simulink model "gm_soc_dvbs2_fpga"  (R2025b)
settings: Solver=VariableStepAuto  StartTime=0.0  StopTime=10.0  RelTol=1e-3
InitFcn:
  | soc_dvbs2_init;
undefined symbols (not defined in the file or in its folder): Add, coefficientsLog, coefficientsSqrt1, coefficientsSqrt2, dataBits, Deinterleaver, designMultirateFIR, noisePow, Shift, Short, soc_dvbs2_designFIRFilter, soc_dvbs2_txPacketBits, syncWord, txDataOut, txFiltCoeff, XData
libraries: simulink x304, hdlsllib x265, dspsigops x15, dsphdlfiltering2 x8, hdlmdlgenlib x6, dsphdlsigops2 x5, commseqgen3 x5, dsphdlmathfun2 x3, hwlogicconnlib x2, whdledac x2, commhdlcrc x2, whdlutilities x1
(part 34 of 36)

== system gm_soc_dvbs2_fpga/DVBS2/DVBS2 TxRx/DVB-S2 HDL Receiver/Synchronizer and PL Header Decoder/Time Frequency and Coarse Phase Synchronizer/Fine Frequency Synchronizer/Modified L and R Algorithm/L and R Algorithm 18 point/Compute R(m) for 1 to 6/Compute R(m)_1 ==
  z : Inport  OutDataTypeStr=fixdt(1, 16, 11)  PortDimensions=1  SampleTime=2.5e-07
      settings: SignalType=complex
  zvalid : Inport  Port=2  OutDataTypeStr=boolean  PortDimensions=1  SampleTime=2.5e-07
  Add3 : Sum  OutDataTypeStr=fixdt(1, 33, 22)  AccumDataTypeStr=fixdt(1, 34, 22)  SampleTime=2.5e-07
  Compare To Constant : simulink/Logic and Bit Operations/Compare To Constant  relop=>=  const="fi(0,0,6,0,\"hex\",\"01\")"  OutDataTypeStr=boolean
  Compare To Constant2 : simulink/Logic and Bit Operations/Compare To Constant  relop===  const="fi(0,0,6,0,\"hex\",\"23\")"  OutDataTypeStr=boolean
  Complex Multiplier : Subsystem
  Delay{,1..2,7..9,11..12,14..15} (10 alike) : Delay  DelayLength=double(1)  InitialCondition=0  SampleTime=2.5e-07
  Delay{3..6,10,13,16..26} (17 alike) : Delay  DelayLength=double(2)  InitialCondition=0  SampleTime=2.5e-07
  Delay{27..30} (4 alike) : Delay  DelayLength=double(8)  InitialCondition=0  SampleTime=2.5e-07
  Gain : Gain  Gain="fi(0,0,16,21,\"hex\",\"ea0f\")"  ParamDataTypeStr=fixdt(0, 16, 21)  OutDataTypeStr=fixdt(1, 33, 22)  SampleTime=2.5e-07
  HDL Counter : hdlsllib/Sources/HDL Counter  CountType=Count limited  CountInit=0  CountStep=1  CountMax=N-1  CountFromType=Initial value  CountFrom=0  CountResetPort=off  CountLoadPort=off  CountEnbPort=on  CountDirPort=off  CountHitOutputPort=off  CountDataType=Unsigned  CountWordLen=nextpow2(N-1)  CountFracLen=0  CountSampTime=1
  Logical Operator : Logic  AllPortsSameDT=off  OutDataTypeStr=boolean  SampleTime=2.5e-07
  Logical Operator1 : Logic  AllPortsSameDT=off  OutDataTypeStr=boolean  SampleTime=2.5e-07
  Math Function : Math  Operator=conj  OutDataTypeStr=fixdt(1, 16, 11)
  Unit Delay Enabled Resettable Synchronous : hdlsllib/Discrete/Unit Delay Enabled Resettable Synchronous  InitialCondition=double(0)  SampleTime=-1
  Unit Delay Enabled Synchronous : hdlsllib/Discrete/Unit Delay Enabled Synchronous  InitialCondition=double(0)  SampleTime=-1
  Out1 : Outport  SampleTime=2.5e-07
  wires:
  zvalid/1 -> Delay14/1
  Logical Operator1/1 -> Delay23/1
  Delay10/1 -> Delay27/1
  Delay21/1 -> Gain/1
  Delay14/1 -> Delay15/1, HDL Counter/1, Delay9/1
  Delay9/1 -> Delay10/1
  HDL Counter/1 -> Delay12/1, Delay11/1
  Delay11/1 -> Delay5/1
  Delay22/1 -> Add3/2
  Delay15/1 -> Delay16/1
  z/1 -> Delay2/1
  Delay12/1 -> Delay6/1
  Delay16/1 -> Delay30/1
  Delay2/1 -> Delay7/1, Delay/1
  Delay27/1 -> Delay17/1
  Delay5/1 -> Delay28/1
  Delay6/1 -> Delay29/1
  Complex Multiplier/1(Out1) -> Delay13/1
  Delay7/1 -> Delay3/1
  Delay/1 -> Math Function/1
  Delay28/1 -> Compare To Constant/1
  Delay29/1 -> Compare To Constant2/1
  Delay30/1 -> Delay20/1
  Delay19/1 -> Logical Operator/1
  Math Function/1 -> Delay8/1
  Delay1/1 -> Unit Delay Enabled Synchronous/2, Unit Delay Enabled Resettable Synchronous/3
  Delay17/1 -> Logical Operator1/1
  Delay13/1 -> Delay21/1
  Compare To Constant2/1 -> Delay19/1
  Compare To Constant/1 -> Delay18/1
  Delay3/1 -> Complex Multiplier/1(In1)
  Delay8/1 -> Delay4/1
  Delay18/1 -> Logical Operator1/2
  Delay20/1 -> Logical Operator/2
  Delay4/1 -> Complex Multiplier/2(In2)
  Logical Operator/1 -> Delay25/1
  Delay24/1 -> Unit Delay Enabled Resettable Synchronous/2
  Delay23/1 -> Delay24/1
  Delay25/1 -> Delay26/1
  Delay26/1 -> Delay1/1
  Gain/1 -> Delay22/1
  Unit Delay Enabled Resettable Synchronous/1 -> Unit Delay Enabled Synchronous/1, Add3/1
  Unit Delay Enabled Synchronous/1 -> Out1/1
  Add3/1 -> Unit Delay Enabled Resettable Synchronous/1

== system gm_soc_dvbs2_fpga/DVBS2/DVBS2 TxRx/DVB-S2 HDL Receiver/Synchronizer and PL Header Decoder/Time Frequency and Coarse Phase Synchronizer/Fine Frequency Synchronizer/Modified L and R Algorithm/L and R Algorithm 18 point/Compute R(m) for 1 to 6/Compute R(m)_2 ==
  z : Inport  OutDataTypeStr=fixdt(1, 16, 11)  PortDimensions=1  SampleTime=2.5e-07
      settings: SignalType=complex
  zvalid : Inport  Port=2  OutDataTypeStr=boolean  PortDimensions=1  SampleTime=2.5e-07
  Add3 : Sum  OutDataTypeStr=fixdt(1, 33, 22)  AccumDataTypeStr=fixdt(1, 34, 22)  SampleTime=2.5e-07
  Compare To Constant : simulink/Logic and Bit Operations/Compare To Constant  relop=>=  const="fi(0,0,6,0,\"hex\",\"02\")"  OutDataTypeStr=boolean
  Compare To Constant2 : simulink/Logic and Bit Operations/Compare To Constant  relop===  const="fi(0,0,6,0,\"hex\",\"23\")"  OutDataTypeStr=boolean
  Complex Multiplier : Subsystem
  Delay{,3..6,10,13,16..26} (18 alike) : Delay  DelayLength=double(2)  InitialCondition=0  SampleTime=2.5e-07
  Delay{1..2,7..9,11..12,14..15} (9 alike) : Delay  DelayLength=double(1)  InitialCondition=0  SampleTime=2.5e-07
  Delay{27..30} (4 alike) : Delay  DelayLength=double(8)  InitialCondition=0  SampleTime=2.5e-07
  Gain : Gain  Gain="fi(0,0,16,21,\"hex\",\"f0f1\")"  ParamDataTypeStr=fixdt(0, 16, 21)  OutDataTypeStr=fixdt(1, 33, 22)  SampleTime=2.5e-07
  HDL Counter : hdlsllib/Sources/HDL Counter  CountType=Count limited  CountInit=0  CountStep=1  CountMax=N-1  CountFromType=Initial value  CountFrom=0  CountResetPort=off  CountLoadPort=off  CountEnbPort=on  CountDirPort=off  CountHitOutputPort=off  CountDataType=Unsigned  CountWordLen=nextpow2(N-1)  CountFracLen=0  CountSampTime=1
  Logical Operator : Logic  AllPortsSameDT=off  OutDataTypeStr=boolean  SampleTime=2.5e-07
  Logical Operator1 : Logic  AllPortsSameDT=off  OutDataTypeStr=boolean  SampleTime=2.5e-07
  Math Function : Math  Operator=conj  OutDataTypeStr=fixdt(1, 16, 11)
  Unit Delay Enabled Resettable Synchronous : hdlsllib/Discrete/Unit Delay Enabled Resettable Synchronous  InitialCondition=double(0)  SampleTime=-1
  Unit Delay Enabled Synchronous : hdlsllib/Discrete/Unit Delay Enabled Synchronous  InitialCondition=double(0)  SampleTime=-1
  Out1 : Outport  SampleTime=2.5e-07
  wires:
  Delay23/1 -> Delay24/1
  zvalid/1 -> Delay14/1
  Delay10/1 -> Delay27/1
  Delay14/1 -> Delay9/1, Delay15/1, HDL Counter/1
  Delay17/1 -> Logical Operator1/1
  Delay9/1 -> Delay10/1
  HDL Counter/1 -> Delay11/1, Delay12/1
  z/1 -> Delay2/1
  Add3/1 -> Unit Delay Enabled Resettable Synchronous/1
  Delay22/1 -> Add3/2
  Delay15/1 -> Delay16/1
  Delay11/1 -> Delay5/1
  Delay12/1 -> Delay6/1
  Delay2/1 -> Delay7/1, Delay/1
  Delay27/1 -> Delay17/1
  Delay5/1 -> Delay28/1
  Delay6/1 -> Delay29/1
  Delay16/1 -> Delay30/1
  Delay/1 -> Math Function/1
  Delay28/1 -> Compare To Constant/1
  Delay29/1 -> Compare To Constant2/1
  Delay7/1 -> Delay3/1
  Math Function/1 -> Delay8/1
  Compare To Constant2/1 -> Delay19/1
  Compare To Constant/1 -> Delay18/1
  Delay30/1 -> Delay20/1
  Delay3/1 -> Complex Multiplier/1(In1)
  Delay8/1 -> Delay4/1
  Logical Operator1/1 -> Delay23/1
  Delay18/1 -> Logical Operator1/2
  Unit Delay Enabled Resettable Synchronous/1 -> Unit Delay Enabled Synchronous/1, Add3/1
  Delay19/1 -> Logical Operator/1
  Delay20/1 -> Logical Operator/2
  Delay4/1 -> Complex Multiplier/2(In2)
  Logical Operator/1 -> Delay25/1
  Complex Multiplier/1(Out1) -> Delay13/1
  Delay25/1 -> Delay26/1
  Delay13/1 -> Delay21/1
  Delay26/1 -> Delay1/1
  Delay21/1 -> Gain/1
  Delay24/1 -> Unit Delay Enabled Resettable Synchronous/2
  Delay1/1 -> Unit Delay Enabled Synchronous/2, Unit Delay Enabled Resettable Synchronous/3
  Gain/1 -> Delay22/1
  Unit Delay Enabled Synchronous/1 -> Out1/1

== system gm_soc_dvbs2_fpga/DVBS2/DVBS2 TxRx/DVB-S2 HDL Receiver/Synchronizer and PL Header Decoder/Time Frequency and Coarse Phase Synchronizer/Fine Frequency Synchronizer/Modified L and R Algorithm/L and R Algorithm 18 point/Compute R(m) for 1 to 6/Compute R(m)_3 ==
  z : Inport  OutDataTypeStr=fixdt(1, 16, 11)  PortDimensions=1  SampleTime=2.5e-07
      settings: SignalType=complex
  zvalid : Inport  Port=2  OutDataTypeStr=boolean  PortDimensions=1  SampleTime=2.5e-07
  Add3 : Sum  OutDataTypeStr=fixdt(1, 33, 22)  AccumDataTypeStr=fixdt(1, 34, 22)  SampleTime=2.5e-07
  Compare To Constant : simulink/Logic and Bit Operations/Compare To Constant  relop=>=  const="fi(0,0,6,0,\"hex\",\"03\")"  OutDataTypeStr=boolean
  Compare To Constant2 : simulink/Logic and Bit Operations/Compare To Constant  relop===  const="fi(0,0,6,0,\"hex\",\"23\")"  OutDataTypeStr=boolean
  Complex Multiplier : Subsystem
  Delay : Delay  DelayLength=double(3)  InitialCondition=0  SampleTime=2.5e-07
  Delay{1..2,7..9,11..12,14..15} (9 alike) : Delay  DelayLength=double(1)  InitialCondition=0  SampleTime=2.5e-07
  Delay{3..6,10,13,16..26} (17 alike) : Delay  DelayLength=double(2)  InitialCondition=0  SampleTime=2.5e-07
  Delay{27..30} (4 alike) : Delay  DelayLength=double(8)  InitialCondition=0  SampleTime=2.5e-07
  Gain : Gain  Gain="fi(0,0,16,21,\"hex\",\"f83e\")"  ParamDataTypeStr=fixdt(0, 16, 21)  OutDataTypeStr=fixdt(1, 33, 22)  SampleTime=2.5e-07
  HDL Counter : hdlsllib/Sources/HDL Counter  CountType=Count limited  CountInit=0  CountStep=1  CountMax=N-1  CountFromType=Initial value  CountFrom=0  CountResetPort=off  CountLoadPort=off  CountEnbPort=on  CountDirPort=off  CountHitOutputPort=off  CountDataType=Unsigned  CountWordLen=nextpow2(N-1)  CountFracLen=0  CountSampTime=1
  Logical Operator : Logic  AllPortsSameDT=off  OutDataTypeStr=boolean  SampleTime=2.5e-07
  Logical Operator1 : Logic  AllPortsSameDT=off  OutDataTypeStr=boolean  SampleTime=2.5e-07
  Math Function : Math  Operator=conj  OutDataTypeStr=fixdt(1, 16, 11)
  Unit Delay Enabled Resettable Synchronous : hdlsllib/Discrete/Unit Delay Enabled Resettable Synchronous  InitialCondition=double(0)  SampleTime=-1
  Unit Delay Enabled Synchronous : hdlsllib/Discrete/Unit Delay Enabled Synchronous  InitialCondition=double(0)  SampleTime=-1
  Out1 : Outport  SampleTime=2.5e-07
  wires:
  Logical Operator/1 -> Delay25/1
  zvalid/1 -> Delay14/1
  Delay10/1 -> Delay27/1
  Delay21/1 -> Gain/1
  Delay14/1 -> Delay15/1, HDL Counter/1, Delay9/1
  Delay9/1 -> Delay10/1
  HDL Counter/1 -> Delay12/1, Delay11/1
  Delay11/1 -> Delay5/1
  Add3/1 -> Unit Delay Enabled Resettable Synchronous/1
  Delay19/1 -> Logical Operator/1
  z/1 -> Delay2/1
  Delay22/1 -> Add3/2
  Delay15/1 -> Delay16/1
  Delay12/1 -> Delay6/1
  Delay16/1 -> Delay30/1
  Delay2/1 -> Delay/1, Delay7/1
  Delay27/1 -> Delay17/1
  Delay5/1 -> Delay28/1
  Delay6/1 -> Delay29/1
  Delay7/1 -> Delay3/1
  Delay23/1 -> Delay24/1
  Delay/1 -> Math Function/1
  Delay28/1 -> Compare To Constant/1
  Delay29/1 -> Compare To Constant2/1
  Delay30/1 -> Delay20/1
  Math Function/1 -> Delay8/1
  Delay1/1 -> Unit Delay Enabled Synchronous/2, Unit Delay Enabled Resettable Synchronous/3
  Compare To Constant2/1 -> Delay19/1
  Compare To Constant/1 -> Delay18/1
  Delay17/1 -> Logical Operator1/1
  Delay3/1 -> Complex Multiplier/1(In1)
  Delay8/1 -> Delay4/1
  Delay18/1 -> Logical Operator1/2
  Delay20/1 -> Logical Operator/2
  Delay4/1 -> Complex Multiplier/2(In2)
  Logical Operator1/1 -> Delay23/1
  Complex Multiplier/1(Out1) -> Delay13/1
  Delay25/1 -> Delay26/1
  Delay13/1 -> Delay21/1
  Delay26/1 -> Delay1/1
  Delay24/1 -> Unit Delay Enabled Resettable Synchronous/2
  Gain/1 -> Delay22/1
  Unit Delay Enabled Resettable Synchronous/1 -> Unit Delay Enabled Synchronous/1, Add3/1
  Unit Delay Enabled Synchronous/1 -> Out1/1

== system gm_soc_dvbs2_fpga/DVBS2/DVBS2 TxRx/DVB-S2 HDL Receiver/Synchronizer and PL Header Decoder/Time Frequency and Coarse Phase Synchronizer/Fine Frequency Synchronizer/Modified L and R Algorithm/L and R Algorithm 18 point/Compute R(m) for 1 to 6/Compute R(m)_4 ==
  z : Inport  OutDataTypeStr=fixdt(1, 16, 11)  PortDimensions=1  SampleTime=2.5e-07
      settings: SignalType=complex
  zvalid : Inport  Port=2  OutDataTypeStr=boolean  PortDimensions=1  SampleTime=2.5e-07
  Add3 : Sum  OutDataTypeStr=fixdt(1, 33, 22)  AccumDataTypeStr=fixdt(1, 34, 22)  SampleTime=2.5e-07
  Compare To Constant : simulink/Logic and Bit Operations/Compare To Constant  relop=>=  const="fi(0,0,6,0,\"hex\",\"04\")"  OutDataTypeStr=boolean
  Compare To Constant2 : simulink/Logic and Bit Operations/Compare To Constant  relop===  const="fi(0,0,6,0,\"hex\",\"23\")"  OutDataTypeStr=boolean
  Complex Multiplier : Subsystem
  Delay : Delay  DelayLength=double(4)  InitialCondition=0  SampleTime=2.5e-07
  Delay{1..2,7..9,11..12,14..15} (9 alike) : Delay  DelayLength=double(1)  InitialCondition=0  SampleTime=2.5e-07
  Delay{3..6,10,13,16..26} (17 alike) : Delay  DelayLength=double(2)  InitialCondition=0  SampleTime=2.5e-07
  Delay{27..30} (4 alike) : Delay  DelayLength=double(8)  InitialCondition=0  SampleTime=2.5e-07
  Gain : Gain  Gain="fi(0,0,16,20,\"hex\",\"8000\")"  ParamDataTypeStr=fixdt(0, 16, 20)  OutDataTypeStr=fixdt(1, 33, 22)  SampleTime=2.5e-07
  HDL Counter : hdlsllib/Sources/HDL Counter  CountType=Count limited  CountInit=0  CountStep=1  CountMax=N-1  CountFromType=Initial value  CountFrom=0  CountResetPort=off  CountLoadPort=off  CountEnbPort=on  CountDirPort=off  CountHitOutputPort=off  CountDataType=Unsigned  CountWordLen=nextpow2(N-1)  CountFracLen=0  CountSampTime=1
  Logical Operator : Logic  AllPortsSameDT=off  OutDataTypeStr=boolean  SampleTime=2.5e-07
  Logical Operator1 : Logic  AllPortsSameDT=off  OutDataTypeStr=boolean  SampleTime=2.5e-07
  Math Function : Math  Operator=conj  OutDataTypeStr=fixdt(1, 16, 11)
  Unit Delay Enabled Resettable Synchronous : hdlsllib/Discrete/Unit Delay Enabled Resettable Synchronous  InitialCondition=double(0)  SampleTime=-1
  Unit Delay Enabled Synchronous : hdlsllib/Discrete/Unit Delay Enabled Synchronous  InitialCondition=double(0)  SampleTime=-1
  Out1 : Outport  SampleTime=2.5e-07
  wires:
  Math Function/1 -> Delay8/1
  zvalid/1 -> Delay14/1
  Delay10/1 -> Delay27/1
  Delay14/1 -> Delay9/1, Delay15/1, HDL Counter/1
  Delay9/1 -> Delay10/1
  HDL Counter/1 -> Delay12/1, Delay11/1
  Delay11/1 -> Delay5/1
  Delay15/1 -> Delay16/1
  z/1 -> Delay2/1
  Delay12/1 -> Delay6/1
  Delay2/1 -> Delay7/1, Delay/1
  Delay27/1 -> Delay17/1
  Delay5/1 -> Delay28/1
  Delay6/1 -> Delay29/1
  Delay16/1 -> Delay30/1
  Delay/1 -> Math Function/1
  Delay28/1 -> Compare To Constant/1
  Delay29/1 -> Compare To Constant2/1
  Delay7/1 -> Delay3/1
  Delay21/1 -> Gain/1
  Compare To Constant2/1 -> Delay19/1
  Compare To Constant/1 -> Delay18/1
  Delay30/1 -> Delay20/1
  Delay3/1 -> Complex Multiplier/1(In1)
  Delay8/1 -> Delay4/1
  Delay1/1 -> Unit Delay Enabled Synchronous/2, Unit Delay Enabled Resettable Synchronous/3
  Delay17/1 -> Logical Operator1/1
  Complex Multiplier/1(Out1) -> Delay13/1
  Delay18/1 -> Logical Operator1/2
  Logical Operator1/1 -> Delay23/1
  Delay19/1 -> Logical Operator/1
  Delay20/1 -> Logical Operator/2
  Delay4/1 -> Complex Multiplier/2(In2)
  Logical Operator/1 -> Delay25/1
  Delay25/1 -> Delay26/1
  Delay13/1 -> Delay21/1
  Delay23/1 -> Delay24/1
  Delay26/1 -> Delay1/1
  Delay24/1 -> Unit Delay Enabled Resettable Synchronous/2
  Gain/1 -> Delay22/1
  Unit Delay Enabled Resettable Synchronous/1 -> Unit Delay Enabled Synchronous/1, Add3/1
  Delay22/1 -> Add3/2
  Unit Delay Enabled Synchronous/1 -> Out1/1
  Add3/1 -> Unit Delay Enabled Resettable Synchronous/1

== system gm_soc_dvbs2_fpga/DVBS2/DVBS2 TxRx/DVB-S2 HDL Receiver/Synchronizer and PL Header Decoder/Time Frequency and Coarse Phase Synchronizer/Fine Frequency Synchronizer/Modified L and R Algorithm/L and R Algorithm 18 point/Compute R(m) for 1 to 6/Compute R(m)_5 ==
  z : Inport  OutDataTypeStr=fixdt(1, 16, 11)  PortDimensions=1  SampleTime=2.5e-07
      settings: SignalType=complex
  zvalid : Inport  Port=2  OutDataTypeStr=boolean  PortDimensions=1  SampleTime=2.5e-07
  Add3 : Sum  OutDataTypeStr=fixdt(1, 33, 22)  AccumDataTypeStr=fixdt(1, 34, 22)  SampleTime=2.5e-07
  Compare To Constant : simulink/Logic and Bit Operations/Compare To Constant  relop=>=  const="fi(0,0,6,0,\"hex\",\"05\")"  OutDataTypeStr=boolean
  Compare To Constant2 : simulink/Logic and Bit Operations/Compare To Constant  relop===  const="fi(0,0,6,0,\"hex\",\"23\")"  OutDataTypeStr=boolean
  Complex Multiplier : Subsystem
  Delay : Delay  DelayLength=double(5)  InitialCondition=0  SampleTime=2.5e-07
  Delay{1..2,7..9,11..12,14..15} (9 alike) : Delay  DelayLength=double(1)  InitialCondition=0  SampleTime=2.5e-07
  Delay{3..6,10,13,16..26} (17 alike) : Delay  DelayLength=double(2)  InitialCondition=0  SampleTime=2.5e-07
  Delay{27..30} (4 alike) : Delay  DelayLength=double(8)  InitialCondition=0  SampleTime=2.5e-07
  Gain : Gain  Gain="fi(0,0,16,20,\"hex\",\"8421\")"  ParamDataTypeStr=fixdt(0, 16, 20)  OutDataTypeStr=fixdt(1, 33, 22)  SampleTime=2.5e-07
  HDL Counter : hdlsllib/Sources/HDL Counter  CountType=Count limited  CountInit=0  CountStep=1  CountMax=N-1  CountFromType=Initial value  CountFrom=0  CountResetPort=off  CountLoadPort=off  CountEnbPort=on  CountDirPort=off  CountHitOutputPort=off  CountDataType=Unsigned  CountWordLen=nextpow2(N-1)  CountFracLen=0  CountSampTime=1
  Logical Operator : Logic  AllPortsSameDT=off  OutDataTypeStr=boolean  SampleTime=2.5e-07
  Logical Operator1 : Logic  AllPortsSameDT=off  OutDataTypeStr=boolean  SampleTime=2.5e-07
  Math Function : Math  Operator=conj  OutDataTypeStr=fixdt(1, 16, 11)
  Unit Delay Enabled Resettable Synchronous : hdlsllib/Discrete/Unit Delay Enabled Resettable Synchronous  InitialCondition=double(0)  SampleTime=-1
  Unit Delay Enabled Synchronous : hdlsllib/Discrete/Unit Delay Enabled Synchronous  InitialCondition=double(0)  SampleTime=-1
  Out1 : Outport  SampleTime=2.5e-07
  wires:
  Delay12/1 -> Delay6/1
  Delay21/1 -> Gain/1
  Logical Operator/1 -> Delay25/1
  Delay14/1 -> Delay9/1, Delay15/1, HDL Counter/1
  Delay10/1 -> Delay27/1
  zvalid/1 -> Delay14/1
  Delay9/1 -> Delay10/1
  Unit Delay Enabled Synchronous/1 -> Out1/1
  HDL Counter/1 -> Delay12/1, Delay11/1
  Math Function/1 -> Delay8/1
  Delay11/1 -> Delay5/1
  Unit Delay Enabled Resettable Synchronous/1 -> Unit Delay Enabled Synchronous/1, Add3/1
  Delay19/1 -> Logical Operator/1
  z/1 -> Delay2/1
  Add3/1 -> Unit Delay Enabled Resettable Synchronous/1
  Delay22/1 -> Add3/2
  Delay15/1 -> Delay16/1
  Delay16/1 -> Delay30/1
  Complex Multiplier/1(Out1) -> Delay13/1
  Delay2/1 -> Delay7/1, Delay/1
  Delay5/1 -> Delay28/1
  Delay6/1 -> Delay29/1
  Delay30/1 -> Delay20/1
  Delay23/1 -> Delay24/1
  Delay/1 -> Math Function/1
  Delay28/1 -> Compare To Constant/1
  Delay29/1 -> Compare To Constant2/1
  Delay7/1 -> Delay3/1
  Delay27/1 -> Delay17/1
  Compare To Constant/1 -> Delay18/1
  Delay20/1 -> Logical Operator/2
  Compare To Constant2/1 -> Delay19/1
  Delay3/1 -> Complex Multiplier/1(In1)
  Delay8/1 -> Delay4/1
  Delay1/1 -> Unit Delay Enabled Synchronous/2, Unit Delay Enabled Resettable Synchronous/3
  Delay17/1 -> Logical Operator1/1
  Logical Operator1/1 -> Delay23/1
  Delay18/1 -> Logical Operator1/2
  Delay4/1 -> Complex Multiplier/2(In2)
  Delay25/1 -> Delay26/1
  Delay13/1 -> Delay21/1
  Delay26/1 -> Delay1/1
  Delay24/1 -> Unit Delay Enabled Resettable Synchronous/2
  Gain/1 -> Delay22/1

== system gm_soc_dvbs2_fpga/DVBS2/DVBS2 TxRx/DVB-S2 HDL Receiver/Synchronizer and PL Header Decoder/Time Frequency and Coarse Phase Synchronizer/Fine Frequency Synchronizer/Modified L and R Algorithm/L and R Algorithm 18 point/Compute R(m) for 1 to 6/Compute R(m)_6 ==
  z : Inport  OutDataTypeStr=fixdt(1, 16, 11)  PortDimensions=1  SampleTime=2.5e-07
      settings: SignalType=complex
  zvalid : Inport  Port=2  OutDataTypeStr=boolean  PortDimensions=1  SampleTime=2.5e-07
  Add3 : Sum  OutDataTypeStr=fixdt(1, 33, 22)  AccumDataTypeStr=fixdt(1, 34, 22)  SampleTime=2.5e-07
  Compare To Constant : simulink/Logic and Bit Operations/Compare To Constant  relop=>=  const="fi(0,0,6,0,\"hex\",\"06\")"  OutDataTypeStr=boolean
  Compare To Constant2 : simulink/Logic and Bit Operations/Compare To Constant  relop===  const="fi(0,0,6,0,\"hex\",\"23\")"  OutDataTypeStr=boolean
  Complex Multiplier : Subsystem
  Delay : Delay  DelayLength=double(6)  InitialCondition=0  SampleTime=2.5e-07
  Delay{1..2,7..9,11..12,14..15} (9 alike) : Delay  DelayLength=double(1)  InitialCondition=0  SampleTime=2.5e-07
  Delay{3..6,10,13,16..26} (17 alike) : Delay  DelayLength=double(2)  InitialCondition=0  SampleTime=2.5e-07
  Delay{27..30} (4 alike) : Delay  DelayLength=double(8)  InitialCondition=0  SampleTime=2.5e-07
  Gain : Gain  Gain="fi(0,0,16,20,\"hex\",\"8889\")"  ParamDataTypeStr=fixdt(0, 16, 20)  OutDataTypeStr=fixdt(1, 33, 22)  SampleTime=2.5e-07
  HDL Counter : hdlsllib/Sources/HDL Counter  CountType=Count limited  CountInit=0  CountStep=1  CountMax=N-1  CountFromType=Initial value  CountFrom=0  CountResetPort=off  CountLoadPort=off  CountEnbPort=on  CountDirPort=off  CountHitOutputPort=off  CountDataType=Unsigned  CountWordLen=nextpow2(N-1)  CountFracLen=0  CountSampTime=1
  Logical Operator : Logic  AllPortsSameDT=off  OutDataTypeStr=boolean  SampleTime=2.5e-07
  Logical Operator1 : Logic  AllPortsSameDT=off  OutDataTypeStr=boolean  SampleTime=2.5e-07
  Math Function : Math  Operator=conj  OutDataTypeStr=fixdt(1, 16, 11)
  Unit Delay Enabled Resettable Synchronous : hdlsllib/Discrete/Unit Delay Enabled Resettable Synchronous  InitialCondition=double(0)  SampleTime=-1
  Unit Delay Enabled Synchronous : hdlsllib/Discrete/Unit Delay Enabled Synchronous  InitialCondition=double(0)  SampleTime=-1
  Out1 : Outport  SampleTime=2.5e-07
  wires:
  Delay23/1 -> Delay24/1
  zvalid/1 -> Delay14/1
  Delay12/1 -> Delay6/1
  Delay14/1 -> Delay9/1, HDL Counter/1, Delay15/1
  Delay9/1 -> Delay10/1
  HDL Counter/1 -> Delay12/1, Delay11/1
  Delay11/1 -> Delay5/1
  Delay15/1 -> Delay16/1
  z/1 -> Delay2/1
  Delay16/1 -> Delay30/1
  Delay2/1 -> Delay7/1, Delay/1
  Logical Operator1/1 -> Delay23/1
  Delay10/1 -> Delay27/1
  Delay5/1 -> Delay28/1
  Delay6/1 -> Delay29/1
  Delay30/1 -> Delay20/1
  Delay/1 -> Math Function/1
  Delay28/1 -> Compare To Constant/1
  Delay29/1 -> Compare To Constant2/1
  Delay7/1 -> Delay3/1
  Delay19/1 -> Logical Operator/1
  Math Function/1 -> Delay8/1
  Delay27/1 -> Delay17/1
  Delay13/1 -> Delay21/1
  Compare To Constant2/1 -> Delay19/1
  Compare To Constant/1 -> Delay18/1
  Delay3/1 -> Complex Multiplier/1(In1)
  Delay8/1 -> Delay4/1
  Delay1/1 -> Unit Delay Enabled Resettable Synchronous/3, Unit Delay Enabled Synchronous/2
  Delay17/1 -> Logical Operator1/1
  Delay18/1 -> Logical Operator1/2
  Delay20/1 -> Logical Operator/2
  Delay4/1 -> Complex Multiplier/2(In2)
  Logical Operator/1 -> Delay25/1
  Complex Multiplier/1(Out1) -> Delay13/1
  Delay25/1 -> Delay26/1
  Delay26/1 -> Delay1/1
  Delay21/1 -> Gain/1
  Delay24/1 -> Unit Delay Enabled Resettable Synchronous/2
  Gain/1 -> Delay22/1
  Unit Delay Enabled Resettable Synchronous/1 -> Unit Delay Enabled Synchronous/1, Add3/1
  Delay22/1 -> Add3/2
  Unit Delay Enabled Synchronous/1 -> Out1/1
  Add3/1 -> Unit Delay Enabled Resettable Synchronous/1

== system gm_soc_dvbs2_fpga/DVBS2/DVBS2 TxRx/DVB-S2 HDL Receiver/Synchronizer and PL Header Decoder/Time Frequency and Coarse Phase Synchronizer/Fine Frequency Synchronizer/Modified L and R Algorithm/L and R Algorithm 18 point/Compute R(m) for 13 to 18/Compute R(m)_1 ==
  z : Inport  OutDataTypeStr=fixdt(1, 16, 11)  PortDimensions=1  SampleTime=2.5e-07
      settings: SignalType=complex
  zvalid : Inport  Port=2  OutDataTypeStr=boolean  PortDimensions=1  SampleTime=2.5e-07
  Add3 : Sum  OutDataTypeStr=fixdt(1, 33, 22)  AccumDataTypeStr=fixdt(1, 34, 22)  SampleTime=2.5e-07
  Compare To Constant : simulink/Logic and Bit Operations/Compare To Constant  relop=>=  const="fi(0,0,6,0,\"hex\",\"0d\")"  OutDataTypeStr=boolean
  Compare To Constant2 : simulink/Logic and Bit Operations/Compare To Constant  relop===  const="fi(0,0,6,0,\"hex\",\"23\")"  OutDataTypeStr=boolean
  Complex Multiplier : Subsystem
  Delay : Delay  DelayLength=double(13)  InitialCondition=0  SampleTime=2.5e-07
  Delay{1..2,7..9,11..12,14..15} (9 alike) : Delay  DelayLength=double(1)  InitialCondition=0  SampleTime=2.5e-07
  Delay{3..6,10,13,16..26} (17 alike) : Delay  DelayLength=double(2)  InitialCondition=0  SampleTime=2.5e-07
  Delay{27..30} (4 alike) : Delay  DelayLength=double(8)  InitialCondition=0  SampleTime=2.5e-07
  Gain : Gain  Gain="fi(0,0,16,20,\"hex\",\"b216\")"  ParamDataTypeStr=fixdt(0, 16, 20)  OutDataTypeStr=fixdt(1, 33, 22)  SampleTime=2.5e-07
  HDL Counter : hdlsllib/Sources/HDL Counter  CountType=Count limited  CountInit=0  CountStep=1  CountMax=N-1  CountFromType=Initial value  CountFrom=0  CountResetPort=off  CountLoadPort=off  CountEnbPort=on  CountDirPort=off  CountHitOutputPort=off  CountDataType=Unsigned  CountWordLen=nextpow2(N-1)  CountFracLen=0  CountSampTime=1
  Logical Operator : Logic  AllPortsSameDT=off  OutDataTypeStr=boolean  SampleTime=2.5e-07
  Logical Operator1 : Logic  AllPortsSameDT=off  OutDataTypeStr=boolean  SampleTime=2.5e-07
  Math Function : Math  Operator=conj  OutDataTypeStr=fixdt(1, 16, 11)
  Unit Delay Enabled Resettable Synchronous : hdlsllib/Discrete/Unit Delay Enabled Resettable Synchronous  InitialCondition=double(0)  SampleTime=-1
  Unit Delay Enabled Synchronous : hdlsllib/Discrete/Unit Delay Enabled Synchronous  InitialCondition=double(0)  SampleTime=-1
  Out1 : Outport  SampleTime=2.5e-07
  wires:
  Delay12/1 -> Delay6/1
  Delay21/1 -> Gain/1
  Logical Operator1/1 -> Delay23/1
  Delay14/1 -> Delay9/1, Delay15/1, HDL Counter/1
  Delay16/1 -> Delay30/1
  zvalid/1 -> Delay14/1
  Delay9/1 -> Delay10/1
  Gain/1 -> Delay22/1
  HDL Counter/1 -> Delay12/1, Delay11/1
  Unit Delay Enabled Resettable Synchronous/1 -> Unit Delay Enabled Synchronous/1, Add3/1
  Delay11/1 -> Delay5/1
  Add3/1 -> Unit Delay Enabled Resettable Synchronous/1
  Delay22/1 -> Add3/2
  Delay15/1 -> Delay16/1
  Delay1/1 -> Unit Delay Enabled Resettable Synchronous/3, Unit Delay Enabled Synchronous/2
  z/1 -> Delay2/1
  Delay2/1 -> Delay7/1, Delay/1
  Delay10/1 -> Delay27/1
  Delay5/1 -> Delay28/1
  Delay6/1 -> Delay29/1
  Delay/1 -> Math Function/1
  Delay28/1 -> Compare To Constant/1
  Delay29/1 -> Compare To Constant2/1
  Complex Multiplier/1(Out1) -> Delay13/1
  Delay30/1 -> Delay20/1
  Delay7/1 -> Delay3/1
  Delay19/1 -> Logical Operator/1
  Math Function/1 -> Delay8/1
  Delay27/1 -> Delay17/1
  Compare To Constant/1 -> Delay18/1
  Delay13/1 -> Delay21/1
  Compare To Constant2/1 -> Delay19/1
  Delay20/1 -> Logical Operator/2
  Delay8/1 -> Delay4/1
  Delay17/1 -> Logical Operator1/1
  Logical Operator/1 -> Delay25/1
  Delay18/1 -> Logical Operator1/2
  Delay3/1 -> Complex Multiplier/1(In1)
  Delay4/1 -> Complex Multiplier/2(In2)
  Delay23/1 -> Delay24/1
  Delay25/1 -> Delay26/1
  Delay26/1 -> Delay1/1
  Delay24/1 -> Unit Delay Enabled Resettable Synchronous/2
  Unit Delay Enabled Synchronous/1 -> Out1/1

== system gm_soc_dvbs2_fpga/DVBS2/DVBS2 TxRx/DVB-S2 HDL Receiver/Synchronizer and PL Header Decoder/Time Frequency and Coarse Phase Synchronizer/Fine Frequency Synchronizer/Modified L and R Algorithm/L and R Algorithm 18 point/Compute R(m) for 13 to 18/Compute R(m)_2 ==
  z : Inport  OutDataTypeStr=fixdt(1, 16, 11)  PortDimensions=1  SampleTime=2.5e-07
      settings: SignalType=complex
  zvalid : Inport  Port=2  OutDataTypeStr=boolean  PortDimensions=1  SampleTime=2.5e-07
  Add3 : Sum  OutDataTypeStr=fixdt(1, 33, 22)  AccumDataTypeStr=fixdt(1, 34, 22)  SampleTime=2.5e-07
  Compare To Constant : simulink/Logic and Bit Operations/Compare To Constant  relop=>=  const="fi(0,0,6,0,\"hex\",\"0e\")"  OutDataTypeStr=boolean
  Compare To Constant2 : simulink/Logic and Bit Operations/Compare To Constant  relop===  const="fi(0,0,6,0,\"hex\",\"23\")"  OutDataTypeStr=boolean
  Complex Multiplier : Subsystem
  Delay : Delay  DelayLength=double(14)  InitialCondition=0  SampleTime=2.5e-07
  Delay{1..2,7..9,11..12,14..15} (9 alike) : Delay  DelayLength=double(1)  InitialCondition=0  SampleTime=2.5e-07
  Delay{3..6,10,13,16..26} (17 alike) : Delay  DelayLength=double(2)  InitialCondition=0  SampleTime=2.5e-07
  Delay{27..30} (4 alike) : Delay  DelayLength=double(8)  InitialCondition=0  SampleTime=2.5e-07
  Gain : Gain  Gain="fi(0,0,16,20,\"hex\",\"ba2f\")"  ParamDataTypeStr=fixdt(0, 16, 20)  OutDataTypeStr=fixdt(1, 33, 22)  SampleTime=2.5e-07
  HDL Counter : hdlsllib/Sources/HDL Counter  CountType=Count limited  CountInit=0  CountStep=1  CountMax=N-1  CountFromType=Initial value  CountFrom=0  CountResetPort=off  CountLoadPort=off  CountEnbPort=on  CountDirPort=off  CountHitOutputPort=off  CountDataType=Unsigned  CountWordLen=nextpow2(N-1)  CountFracLen=0  CountSampTime=1
  Logical Operator : Logic  AllPortsSameDT=off  OutDataTypeStr=boolean  SampleTime=2.5e-07
  Logical Operator1 : Logic  AllPortsSameDT=off  OutDataTypeStr=boolean  SampleTime=2.5e-07
  Math Function : Math  Operator=conj  OutDataTypeStr=fixdt(1, 16, 11)
  Unit Delay Enabled Resettable Synchronous : hdlsllib/Discrete/Unit Delay Enabled Resettable Synchronous  InitialCondition=double(0)  SampleTime=-1
  Unit Delay Enabled Synchronous : hdlsllib/Discrete/Unit Delay Enabled Synchronous  InitialCondition=double(0)  SampleTime=-1
  Out1 : Outport  SampleTime=2.5e-07
  wires:
  zvalid/1 -> Delay14/1
  Delay10/1 -> Delay27/1
  Logical Operator1/1 -> Delay23/1
  Delay14/1 -> Delay9/1, HDL Counter/1, Delay15/1
  Delay9/1 -> Delay10/1
  HDL Counter/1 -> Delay12/1, Delay11/1
  Delay11/1 -> Delay5/1
  Add3/1 -> Unit Delay Enabled Resettable Synchronous/1
  Delay15/1 -> Delay16/1
  z/1 -> Delay2/1
  Delay12/1 -> Delay6/1
  Delay2/1 -> Delay7/1, Delay/1
  Delay5/1 -> Delay28/1
  Delay6/1 -> Delay29/1
  Delay16/1 -> Delay30/1
  Delay/1 -> Math Function/1
  Delay27/1 -> Delay17/1
  Delay28/1 -> Compare To Constant/1
  Delay29/1 -> Compare To Constant2/1
  Delay7/1 -> Delay3/1
  Delay19/1 -> Logical Operator/1
  Math Function/1 -> Delay8/1
  Delay13/1 -> Delay21/1
  Compare To Constant2/1 -> Delay19/1
  Compare To Constant/1 -> Delay18/1
  Delay30/1 -> Delay20/1
  Delay3/1 -> Complex Multiplier/1(In1)
  Delay8/1 -> Delay4/1
  Delay1/1 -> Unit Delay Enabled Synchronous/2, Unit Delay Enabled Resettable Synchronous/3
  Delay17/1 -> Logical Operator1/1
  Logical Operator/1 -> Delay25/1
  Delay18/1 -> Logical Operator1/2
  Delay20/1 -> Logical Operator/2
  Delay4/1 -> Complex Multiplier/2(In2)
  Delay21/1 -> Gain/1
  Complex Multiplier/1(Out1) -> Delay13/1
  Delay24/1 -> Unit Delay Enabled Resettable Synchronous/2
  Delay23/1 -> Delay24/1
  Delay25/1 -> Delay26/1
  Delay26/1 -> Delay1/1
  Gain/1 -> Delay22/1
  Unit Delay Enabled Resettable Synchronous/1 -> Unit Delay Enabled Synchronous/1, Add3/1
  Delay22/1 -> Add3/2
  Unit Delay Enabled Synchronous/1 -> Out1/1

== system gm_soc_dvbs2_fpga/DVBS2/DVBS2 TxRx/DVB-S2 HDL Receiver/Synchronizer and PL Header Decoder/Time Frequency and Coarse Phase Synchronizer/Fine Frequency Synchronizer/Modified L and R Algorithm/L and R Algorithm 18 point/Compute R(m) for 13 to 18/Compute R(m)_3 ==
  z : Inport  OutDataTypeStr=fixdt(1, 16, 11)  PortDimensions=1  SampleTime=2.5e-07
      settings: SignalType=complex
  zvalid : Inport  Port=2  OutDataTypeStr=boolean  PortDimensions=1  SampleTime=2.5e-07
  Add3 : Sum  OutDataTypeStr=fixdt(1, 33, 22)  AccumDataTypeStr=fixdt(1, 34, 22)  SampleTime=2.5e-07
  Compare To Constant : simulink/Logic and Bit Operations/Compare To Constant  relop=>=  const="fi(0,0,6,0,\"hex\",\"0f\")"  OutDataTypeStr=boolean
  Compare To Constant2 : simulink/Logic and Bit Operations/Compare To Constant  relop===  const="fi(0,0,6,0,\"hex\",\"23\")"  OutDataTypeStr=boolean
  Complex Multiplier : Subsystem
  Delay : Delay  DelayLength=double(15)  InitialCondition=0  SampleTime=2.5e-07
  Delay{1..2,7..9,11..12,14..15} (9 alike) : Delay  DelayLength=double(1)  InitialCondition=0  SampleTime=2.5e-07
  Delay{3..6,10,13,16..26} (17 alike) : Delay  DelayLength=double(2)  InitialCondition=0  SampleTime=2.5e-07
  Delay{27..30} (4 alike) : Delay  DelayLength=double(8)  InitialCondition=0  SampleTime=2.5e-07
  Gain : Gain  Gain="fi(0,0,16,20,\"hex\",\"c30c\")"  ParamDataTypeStr=fixdt(0, 16, 20)  OutDataTypeStr=fixdt(1, 33, 22)  SampleTime=2.5e-07
  HDL Counter : hdlsllib/Sources/HDL Counter  CountType=Count limited  CountInit=0  CountStep=1  CountMax=N-1  CountFromType=Initial value  CountFrom=0  CountResetPort=off  CountLoadPort=off  CountEnbPort=on  CountDirPort=off  CountHitOutputPort=off  CountDataType=Unsigned  CountWordLen=nextpow2(N-1)  CountFracLen=0  CountSampTime=1
  Logical Operator : Logic  AllPortsSameDT=off  OutDataTypeStr=boolean  SampleTime=2.5e-07
  Logical Operator1 : Logic  AllPortsSameDT=off  OutDataTypeStr=boolean  SampleTime=2.5e-07
  Math Function : Math  Operator=conj  OutDataTypeStr=fixdt(1, 16, 11)
  Unit Delay Enabled Resettable Synchronous : hdlsllib/Discrete/Unit Delay Enabled Resettable Synchronous  InitialCondition=double(0)  SampleTime=-1
  Unit Delay Enabled Synchronous : hdlsllib/Discrete/Unit Delay Enabled Synchronous  InitialCondition=double(0)  SampleTime=-1
  Out1 : Outport  SampleTime=2.5e-07
  wires:
  Delay21/1 -> Gain/1
  Delay14/1 -> Delay15/1, Delay9/1, HDL Counter/1
  Logical Operator/1 -> Delay25/1
  zvalid/1 -> Delay14/1
  Delay9/1 -> Delay10/1
  Gain/1 -> Delay22/1
  HDL Counter/1 -> Delay12/1, Delay11/1
  Unit Delay Enabled Resettable Synchronous/1 -> Unit Delay Enabled Synchronous/1, Add3/1
  Delay19/1 -> Logical Operator/1
  z/1 -> Delay2/1
  Delay22/1 -> Add3/2
  Delay15/1 -> Delay16/1
  Delay10/1 -> Delay27/1
  Delay11/1 -> Delay5/1
  Delay12/1 -> Delay6/1
  Delay16/1 -> Delay30/1
  Delay2/1 -> Delay/1, Delay7/1
  Delay5/1 -> Delay28/1
  Delay6/1 -> Delay29/1
  Delay30/1 -> Delay20/1
  Delay7/1 -> Delay3/1
  Delay/1 -> Math Function/1
  Delay27/1 -> Delay17/1
  Delay28/1 -> Compare To Constant/1
  Delay29/1 -> Compare To Constant2/1
  Math Function/1 -> Delay8/1
  Delay1/1 -> Unit Delay Enabled Synchronous/2, Unit Delay Enabled Resettable Synchronous/3
  Compare To Constant2/1 -> Delay19/1
  Compare To Constant/1 -> Delay18/1
  Delay20/1 -> Logical Operator/2
  Delay3/1 -> Complex Multiplier/1(In1)
  Delay8/1 -> Delay4/1
  Delay17/1 -> Logical Operator1/1
  Delay18/1 -> Logical Operator1/2
  Delay4/1 -> Complex Multiplier/2(In2)
  Logical Operator1/1 -> Delay23/1
  Delay23/1 -> Delay24/1
  Complex Multiplier/1(Out1) -> Delay13/1
  Delay25/1 -> Delay26/1
  Delay13/1 -> Delay21/1
  Delay26/1 -> Delay1/1
  Delay24/1 -> Unit Delay Enabled Resettable Synchronous/2
  Unit Delay Enabled Synchronous/1 -> Out1/1
  Add3/1 -> Unit Delay Enabled Resettable Synchronous/1

== system gm_soc_dvbs2_fpga/DVBS2/DVBS2 TxRx/DVB-S2 HDL Receiver/Synchronizer and PL Header Decoder/Time Frequency and Coarse Phase Synchronizer/Fine Frequency Synchronizer/Modified L and R Algorithm/L and R Algorithm 18 point/Compute R(m) for 13 to 18/Compute R(m)_4 ==
  z : Inport  OutDataTypeStr=fixdt(1, 16, 11)  PortDimensions=1  SampleTime=2.5e-07
      settings: SignalType=complex
  zvalid : Inport  Port=2  OutDataTypeStr=boolean  PortDimensions=1  SampleTime=2.5e-07
  Add3 : Sum  OutDataTypeStr=fixdt(1, 33, 22)  AccumDataTypeStr=fixdt(1, 34, 22)  SampleTime=2.5e-07
  Compare To Constant : simulink/Logic and Bit Operations/Compare To Constant  relop=>=  const="fi(0,0,6,0,\"hex\",\"10\")"  OutDataTypeStr=boolean
  Compare To Constant2 : simulink/Logic and Bit Operations/Compare To Constant  relop===  const="fi(0,0,6,0,\"hex\",\"23\")"  OutDataTypeStr=boolean
  Complex Multiplier : Subsystem
  Delay : Delay  DelayLength=double(16)  InitialCondition=0  SampleTime=2.5e-07
  Delay{1..2,7..9,11..12,14..15} (9 alike) : Delay  DelayLength=double(1)  InitialCondition=0  SampleTime=2.5e-07
  Delay{3..6,10,13,16..26} (17 alike) : Delay  DelayLength=double(2)  InitialCondition=0  SampleTime=2.5e-07
  Delay{27..30} (4 alike) : Delay  DelayLength=double(8)  InitialCondition=0  SampleTime=2.5e-07
  Gain : Gain  Gain="fi(0,0,16,20,\"hex\",\"cccd\")"  ParamDataTypeStr=fixdt(0, 16, 20)  OutDataTypeStr=fixdt(1, 33, 22)  SampleTime=2.5e-07
  HDL Counter : hdlsllib/Sources/HDL Counter  CountType=Count limited  CountInit=0  CountStep=1  CountMax=N-1  CountFromType=Initial value  CountFrom=0  CountResetPort=off  CountLoadPort=off  CountEnbPort=on  CountDirPort=off  CountHitOutputPort=off  CountDataType=Unsigned  CountWordLen=nextpow2(N-1)  CountFracLen=0  CountSampTime=1
  Logical Operator : Logic  AllPortsSameDT=off  OutDataTypeStr=boolean  SampleTime=2.5e-07
  Logical Operator1 : Logic  AllPortsSameDT=off  OutDataTypeStr=boolean  SampleTime=2.5e-07
  Math Function : Math  Operator=conj  OutDataTypeStr=fixdt(1, 16, 11)
  Unit Delay Enabled Resettable Synchronous : hdlsllib/Discrete/Unit Delay Enabled Resettable Synchronous  InitialCondition=double(0)  SampleTime=-1
  Unit Delay Enabled Synchronous : hdlsllib/Discrete/Unit Delay Enabled Synchronous  InitialCondition=double(0)  SampleTime=-1
  Out1 : Outport  SampleTime=2.5e-07
  wires:
  Delay10/1 -> Delay27/1
  Delay21/1 -> Gain/1
  Logical Operator/1 -> Delay25/1
  Delay14/1 -> Delay9/1, Delay15/1, HDL Counter/1
  Delay12/1 -> Delay6/1
  zvalid/1 -> Delay14/1
  Delay9/1 -> Delay10/1
  HDL Counter/1 -> Delay12/1, Delay11/1
  Add3/1 -> Unit Delay Enabled Resettable Synchronous/1
  Delay11/1 -> Delay5/1
  Delay1/1 -> Unit Delay Enabled Synchronous/2, Unit Delay Enabled Resettable Synchronous/3
  Delay17/1 -> Logical Operator1/1
  z/1 -> Delay2/1
  Delay22/1 -> Add3/2
  Delay15/1 -> Delay16/1
  Delay16/1 -> Delay30/1
  Delay2/1 -> Delay7/1, Delay/1
  Delay27/1 -> Delay17/1
  Delay5/1 -> Delay28/1
  Delay6/1 -> Delay29/1
  Delay30/1 -> Delay20/1
  Delay7/1 -> Delay3/1
  Delay23/1 -> Delay24/1
  Delay/1 -> Math Function/1
  Delay28/1 -> Compare To Constant/1
  Delay29/1 -> Compare To Constant2/1
  Math Function/1 -> Delay8/1
  Compare To Constant2/1 -> Delay19/1
  Compare To Constant/1 -> Delay18/1
  Delay3/1 -> Complex Multiplier/1(In1)
  Delay8/1 -> Delay4/1
  Logical Operator1/1 -> Delay23/1
  Delay18/1 -> Logical Operator1/2
  Delay19/1 -> Logical Operator/1
  Delay20/1 -> Logical Operator/2
  Delay4/1 -> Complex Multiplier/2(In2)
  Complex Multiplier/1(Out1) -> Delay13/1
  Delay25/1 -> Delay26/1
  Delay13/1 -> Delay21/1
  Delay26/1 -> Delay1/1
  Delay24/1 -> Unit Delay Enabled Resettable Synchronous/2
  Gain/1 -> Delay22/1
  Unit Delay Enabled Resettable Synchronous/1 -> Unit Delay Enabled Synchronous/1, Add3/1
  Unit Delay Enabled Synchronous/1 -> Out1/1

== system gm_soc_dvbs2_fpga/DVBS2/DVBS2 TxRx/DVB-S2 HDL Receiver/Synchronizer and PL Header Decoder/Time Frequency and Coarse Phase Synchronizer/Fine Frequency Synchronizer/Modified L and R Algorithm/L and R Algorithm 18 point/Compute R(m) for 13 to 18/Compute R(m)_5 ==
  z : Inport  OutDataTypeStr=fixdt(1, 16, 11)  PortDimensions=1  SampleTime=2.5e-07
      settings: SignalType=complex
  zvalid : Inport  Port=2  OutDataTypeStr=boolean  PortDimensions=1  SampleTime=2.5e-07
  Add3 : Sum  OutDataTypeStr=fixdt(1, 33, 22)  AccumDataTypeStr=fixdt(1, 34, 22)  SampleTime=2.5e-07
  Compare To Constant : simulink/Logic and Bit Operations/Compare To Constant  relop=>=  const="fi(0,0,6,0,\"hex\",\"11\")"  OutDataTypeStr=boolean
  Compare To Constant2 : simulink/Logic and Bit Operations/Compare To Constant  relop===  const="fi(0,0,6,0,\"hex\",\"23\")"  OutDataTypeStr=boolean
  Complex Multiplier : Subsystem
  Delay : Delay  DelayLength=double(17)  InitialCondition=0  SampleTime=2.5e-07
  Delay{1..2,7..9,11..12,14..15} (9 alike) : Delay  DelayLength=double(1)  InitialCondition=0  SampleTime=2.5e-07
  Delay{3..6,10,13,16..26} (17 alike) : Delay  DelayLength=double(2)  InitialCondition=0  SampleTime=2.5e-07
  Delay{27..30} (4 alike) : Delay  DelayLength=double(8)  InitialCondition=0  SampleTime=2.5e-07
  Gain : Gain  Gain="fi(0,0,16,20,\"hex\",\"d794\")"  ParamDataTypeStr=fixdt(0, 16, 20)  OutDataTypeStr=fixdt(1, 33, 22)  SampleTime=2.5e-07
  HDL Counter : hdlsllib/Sources/HDL Counter  CountType=Count limited  CountInit=0  CountStep=1  CountMax=N-1  CountFromType=Initial value  CountFrom=0  CountResetPort=off  CountLoadPort=off  CountEnbPort=on  CountDirPort=off  CountHitOutputPort=off  CountDataType=Unsigned  CountWordLen=nextpow2(N-1)  CountFracLen=0  CountSampTime=1
  Logical Operator : Logic  AllPortsSameDT=off  OutDataTypeStr=boolean  SampleTime=2.5e-07
  Logical Operator1 : Logic  AllPortsSameDT=off  OutDataTypeStr=boolean  SampleTime=2.5e-07
  Math Function : Math  Operator=conj  OutDataTypeStr=fixdt(1, 16, 11)
  Unit Delay Enabled Resettable Synchronous : hdlsllib/Discrete/Unit Delay Enabled Resettable Synchronous  InitialCondition=double(0)  SampleTime=-1
  Unit Delay Enabled Synchronous : hdlsllib/Discrete/Unit Delay Enabled Synchronous  InitialCondition=double(0)  SampleTime=-1
  Out1 : Outport  SampleTime=2.5e-07
  wires:
  zvalid/1 -> Delay14/1
  Delay10/1 -> Delay27/1
  Logical Operator/1 -> Delay25/1
  Delay14/1 -> Delay9/1, Delay15/1, HDL Counter/1
  Delay9/1 -> Delay10/1
  HDL Counter/1 -> Delay12/1, Delay11/1
  Math Function/1 -> Delay8/1
  z/1 -> Delay2/1
  Delay22/1 -> Add3/2
  Unit Delay Enabled Resettable Synchronous/1 -> Unit Delay Enabled Synchronous/1, Add3/1
  Delay15/1 -> Delay16/1
  Delay11/1 -> Delay5/1
  Delay12/1 -> Delay6/1
  Delay16/1 -> Delay30/1
  Complex Multiplier/1(Out1) -> Delay13/1
  Delay2/1 -> Delay7/1, Delay/1
  Delay27/1 -> Delay17/1
  Delay5/1 -> Delay28/1
  Delay6/1 -> Delay29/1
  Delay7/1 -> Delay3/1
  Delay/1 -> Math Function/1
  Delay28/1 -> Compare To Constant/1
  Delay29/1 -> Compare To Constant2/1
  Delay30/1 -> Delay20/1
  Delay17/1 -> Logical Operator1/1
  Compare To Constant2/1 -> Delay19/1
  Compare To Constant/1 -> Delay18/1
  Delay3/1 -> Complex Multiplier/1(In1)
  Delay8/1 -> Delay4/1
  Delay18/1 -> Logical Operator1/2
  Delay19/1 -> Logical Operator/1
  Delay20/1 -> Logical Operator/2
  Delay4/1 -> Complex Multiplier/2(In2)
  Logical Operator1/1 -> Delay23/1
  Delay25/1 -> Delay26/1
  Delay13/1 -> Delay21/1
  Delay23/1 -> Delay24/1
  Delay26/1 -> Delay1/1
  Delay21/1 -> Gain/1
  Delay24/1 -> Unit Delay Enabled Resettable Synchronous/2
  Delay1/1 -> Unit Delay Enabled Synchronous/2, Unit Delay Enabled Resettable Synchronous/3
  Gain/1 -> Delay22/1
  Unit Delay Enabled Synchronous/1 -> Out1/1
  Add3/1 -> Unit Delay Enabled Resettable Synchronous/1

== system gm_soc_dvbs2_fpga/DVBS2/DVBS2 TxRx/DVB-S2 HDL Receiver/Synchronizer and PL Header Decoder/Time Frequency and Coarse Phase Synchronizer/Fine Frequency Synchronizer/Modified L and R Algorithm/L and R Algorithm 18 point/Compute R(m) for 13 to 18/Compute R(m)_6 ==
  z : Inport  OutDataTypeStr=fixdt(1, 16, 11)  PortDimensions=1  SampleTime=2.5e-07
      settings: SignalType=complex
  zvalid : Inport  Port=2  OutDataTypeStr=boolean  PortDimensions=1  SampleTime=2.5e-07
  Add3 : Sum  OutDataTypeStr=fixdt(1, 33, 22)  AccumDataTypeStr=fixdt(1, 34, 22)  SampleTime=2.5e-07
  Compare To Constant : simulink/Logic and Bit Operations/Compare To Constant  relop=>=  const="fi(0,0,6,0,\"hex\",\"12\")"  OutDataTypeStr=boolean
  Compare To Constant2 : simulink/Logic and Bit Operations/Compare To Constant  relop===  const="fi(0,0,6,0,\"hex\",\"23\")"  OutDataTypeStr=boolean
  Complex Multiplier : Subsystem
  Delay : Delay  DelayLength=double(18)  InitialCondition=0  SampleTime=2.5e-07
  Delay{1..2,7..9,11..12,14..15} (9 alike) : Delay  DelayLength=double(1)  InitialCondition=0  SampleTime=2.5e-07
  Delay{3..6,10,13,16..26} (17 alike) : Delay  DelayLength=double(2)  InitialCondition=0  SampleTime=2.5e-07
  Delay{27..30} (4 alike) : Delay  DelayLength=double(8)  InitialCondition=0  SampleTime=2.5e-07
  Gain : Gain  Gain="fi(0,0,16,20,\"hex\",\"e38e\")"  ParamDataTypeStr=fixdt(0, 16, 20)  OutDataTypeStr=fixdt(1, 33, 22)  SampleTime=2.5e-07
  HDL Counter : hdlsllib/Sources/HDL Counter  CountType=Count limited  CountInit=0  CountStep=1  CountMax=N-1  CountFromType=Initial value  CountFrom=0  CountResetPort=off  CountLoadPort=off  CountEnbPort=on  CountDirPort=off  CountHitOutputPort=off  CountDataType=Unsigned  CountWordLen=nextpow2(N-1)  CountFracLen=0  CountSampTime=1
  Logical Operator : Logic  AllPortsSameDT=off  OutDataTypeStr=boolean  SampleTime=2.5e-07
  Logical Operator1 : Logic  AllPortsSameDT=off  OutDataTypeStr=boolean  SampleTime=2.5e-07
  Math Function : Math  Operator=conj  OutDataTypeStr=fixdt(1, 16, 11)
  Unit Delay Enabled Resettable Synchronous : hdlsllib/Discrete/Unit Delay Enabled Resettable Synchronous  InitialCondition=double(0)  SampleTime=-1
  Unit Delay Enabled Synchronous : hdlsllib/Discrete/Unit Delay Enabled Synchronous  InitialCondition=double(0)  SampleTime=-1
  Out1 : Outport  SampleTime=2.5e-07
  wires:
  zvalid/1 -> Delay14/1
  Delay12/1 -> Delay6/1
  Delay21/1 -> Gain/1
  Logical Operator1/1 -> Delay23/1
  Delay14/1 -> Delay9/1, Delay15/1, HDL Counter/1
  Delay9/1 -> Delay10/1
  HDL Counter/1 -> Delay12/1, Delay11/1
  Delay11/1 -> Delay5/1
  Delay1/1 -> Unit Delay Enabled Synchronous/2, Unit Delay Enabled Resettable Synchronous/3
  Delay17/1 -> Logical Operator1/1
  z/1 -> Delay2/1
  Add3/1 -> Unit Delay Enabled Resettable Synchronous/1
  Delay22/1 -> Add3/2
  Delay15/1 -> Delay16/1
  Delay16/1 -> Delay30/1
  Delay2/1 -> Delay7/1, Delay/1
  Delay10/1 -> Delay27/1
  Delay5/1 -> Delay28/1
  Delay6/1 -> Delay29/1
  Delay30/1 -> Delay20/1
  Delay23/1 -> Delay24/1
  Delay/1 -> Math Function/1
  Delay28/1 -> Compare To Constant/1
  Delay29/1 -> Compare To Constant2/1
  Delay7/1 -> Delay3/1
  Delay19/1 -> Logical Operator/1
  Math Function/1 -> Delay8/1
  Unit Delay Enabled Resettable Synchronous/1 -> Unit Delay Enabled Synchronous/1, Add3/1
  Delay27/1 -> Delay17/1
  Delay13/1 -> Delay21/1
  Compare To Constant2/1 -> Delay19/1
  Compare To Constant/1 -> Delay18/1
  Delay3/1 -> Complex Multiplier/1(In1)
  Delay8/1 -> Delay4/1
  Logical Operator/1 -> Delay25/1
  Delay18/1 -> Logical Operator1/2
  Delay20/1 -> Logical Operator/2
  Delay4/1 -> Complex Multiplier/2(In2)
  Complex Multiplier/1(Out1) -> Delay13/1
  Delay25/1 -> Delay26/1
  Delay26/1 -> Delay1/1
  Delay24/1 -> Unit Delay Enabled Resettable Synchronous/2
  Gain/1 -> Delay22/1
  Unit Delay Enabled Synchronous/1 -> Out1/1
